simulink subsystem "climb_control"  (R2021a)
settings: Solver=VariableStepAuto  StartTime=0.0  StopTime=10.0  RelTol=1e-3
undefined symbols (not defined in the file or in its folder): DiscIntNeverNeededParam, g, ki_climb, kp_climb, m_wet, Nbar_climb, T_max, Ts_climb
settings Model: Creator=EpEp  LastModifiedBy=EpEp

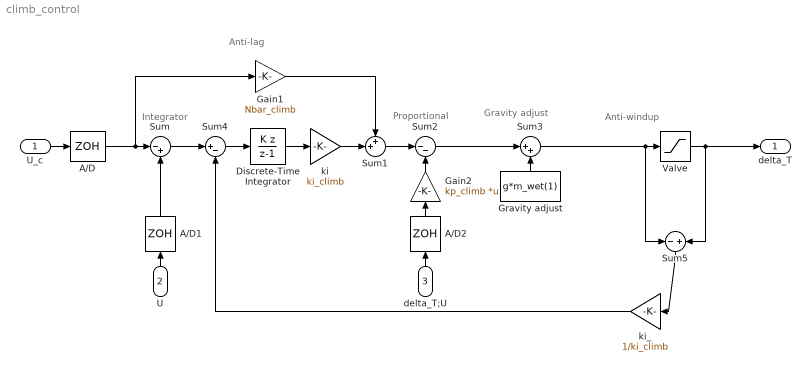
== system climb_control ==
  note: Proportional
  note: Gravity adjust
  note: Integrator
  note: Anti-lag
  note: Anti-windup
  U_c : Inport
  U : Inport  Port=2
  delta_T;U : Inport  Port=3
  A/D : ZeroOrderHold  SampleTime=Ts_climb
  A/D1 : ZeroOrderHold  SampleTime=Ts_climb
  A/D2 : ZeroOrderHold  SampleTime=Ts_climb
  Discrete-Time Integrator : DiscreteIntegrator  IntegratorMethod=Accumulation: Backward Euler  SampleTime=-1  ICPrevOutput=DiscIntNeverNeededParam  ICPrevScaledInput=DiscIntNeverNeededParam
  Gain1 : Gain  Gain=Nbar_climb
  Gain2 : Gain  Gain=kp_climb  Multiplication=Matrix(K*u)
  Gravity adjust : Constant  Value=g*m_wet(1)
  Sum : Sum  Inputs=|-+
  Sum1 : Sum  Inputs=++|
  Sum2 : Sum  Inputs=|--
  Sum3 : Sum  Inputs=|++
  Sum4 : Sum  Inputs=|+-
  Sum5 : Sum  Inputs=-+
  Valve : Saturate  UpperLimit=T_max  LowerLimit=0
  ki : Gain  Gain=ki_climb
  ki_ : Gain  Gain=1/ki_climb
  delta_T : Outport
  wires:
  U_c/1 -> A/D/1
  A/D/1 -> Sum/1, Gain1/1
  Discrete-Time Integrator/1 -> ki/1
  ki/1 -> Sum1/2
  Gain1/1 -> Sum1/1
  Sum1/1 -> Sum2/1
  delta_T;U/1 -> A/D2/1
  A/D1/1 -> Sum/2
  U/1 -> A/D1/1
  Gain2/1 -> Sum2/2
  A/D2/1 -> Gain2/1
  Sum2/1 -> Sum3/1
  Sum3/1 -> Valve/1, Sum5/1
  Valve/1 -> delta_T/1, Sum5/2
  Gravity adjust/1 -> Sum3/2
  Sum4/1 -> Discrete-Time Integrator/1
  Sum/1 -> Sum4/1
  Sum5/1 -> ki_/1
  ki_/1 -> Sum4/2
